simulink model "GDFLIB_FilterIIR2_BAM_FLT"  (Simulink 8.3)
settings: Solver=ode45  StartTime=0.0  StopTime=10.0  RelTol=1e-3
undefined symbols (not defined in the file): fltA1, fltA2, fltB0, fltB1, fltB2
settings Model: Creator=B17364  LastModifiedBy=B17364
settings OptimizationCC: ExpressionDepthLimit=2147483647
settings DebuggingCC: FcnCallInpInsideContextMsg=UseLocalSettings  StrictBusMsg=Warning

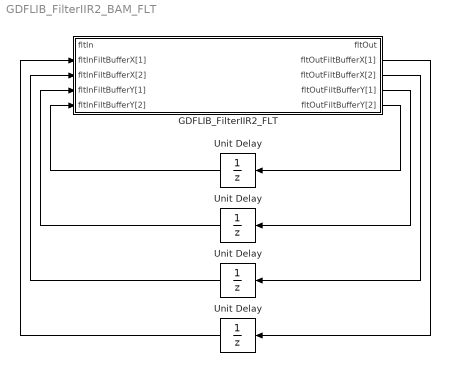
== system GDFLIB_FilterIIR2_BAM_FLT ==
  " Unit Delay" : UnitDelay  SampleTime=-1
  " Unit Delay " : UnitDelay  SampleTime=-1
  GDFLIB_FilterIIR2_FLT : Subsystem  mask(GDFLIB_FilterIIR2){fltB0=fltB0, fltB1=fltB1, fltB2=fltB2, fltA1=fltA1, fltA2=fltA2}
      mask help: Bit accurate model of direct form I second order IIR filter. All parameters as well as input and output are in single precision floating data format.
      mask init:
      | pos = get_param(gcb, 'Position');width = pos(3) - pos(1); height = pos(4) - pos(2);tX=width/2;tY=height*0.9;
      mask Display: color('black');port_label('input',1,'fltIn');port_label('input',2,'fltInFiltBufferX[1]');port_label('input',3,'fltInFiltBufferX[2]');port_label('input',4,'fltInFiltBufferY[1]');port_label('input',5,'fltInFiltBufferY[2]');port_label('output',1,'fltOut');port_label('output',2,'fltOutFiltBufferX[1]');port_label('output',3,'fltOutFiltBufferX[2]');port_label('output',4,'fltOutFiltBufferY[1]');port_label('output',5,'fltOutFiltBufferY[2]');color('black');disp('GDFLIB_FilterIIR2_FLT');color('blue');text(tX,tY, 'BAM', 'horizontalAlignment', 'center');
  Unit Delay : UnitDelay  SampleTime=-1
  "Unit Delay " : UnitDelay  SampleTime=-1
  wires:
  GDFLIB_FilterIIR2_FLT/5(fltOutFiltBufferY[2]) -> Unit Delay/1
  Unit Delay/1 -> GDFLIB_FilterIIR2_FLT/5(fltInFiltBufferY[2])
  GDFLIB_FilterIIR2_FLT/4(fltOutFiltBufferY[1]) -> "Unit Delay "/1
  "Unit Delay "/1 -> GDFLIB_FilterIIR2_FLT/4(fltInFiltBufferY[1])
  GDFLIB_FilterIIR2_FLT/3(fltOutFiltBufferX[2]) -> " Unit Delay"/1
  " Unit Delay"/1 -> GDFLIB_FilterIIR2_FLT/3(fltInFiltBufferX[2])
  GDFLIB_FilterIIR2_FLT/2(fltOutFiltBufferX[1]) -> " Unit Delay "/1
  " Unit Delay "/1 -> GDFLIB_FilterIIR2_FLT/2(fltInFiltBufferX[1])

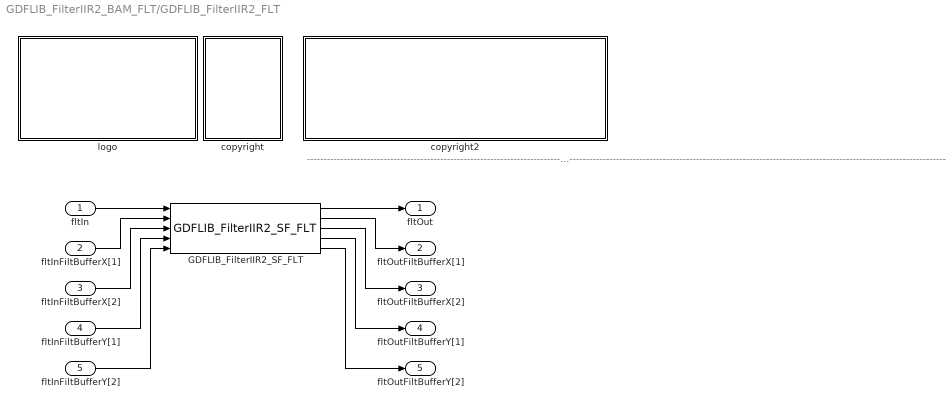
== system GDFLIB_FilterIIR2_BAM_FLT/GDFLIB_FilterIIR2_FLT ==
  note: ---------------------------------------------------------------------------------------------------------------------------------------------------------------------------------------------------
  fltIn : Inport
  fltInFiltBufferX[1] : Inport  Port=2
  fltInFiltBufferX[2] : Inport  Port=3
  fltInFiltBufferY[1] : Inport  Port=4
  fltInFiltBufferY[2] : Inport  Port=5
  GDFLIB_FilterIIR2_SF_FLT : S-Function  FunctionName=GDFLIB_FilterIIR2_SF_FLT  Parameters=fltB0,fltB1,fltB2,fltA1,fltA2  EnableBusSupport=off
  copyright : Subsystem
      mask Display:
      | text(10,90,'FILE:');text(10,75,'DESRIPTION:')
      | text(10,60,'COPYRIGHT:')
      | text(10,45,'VERSION:')
      | text(10,30,'DATE:')
      | text(10,15,'AUTHOR:')
  copyright2 : Subsystem
      mask Display:
      | text(10,90,'GDFLIB_FilterIIR2_BAM_FLT.mdl');text(10,75,'Direct form I second order IIR filter.');text(10,60,'Freescale')
      | text(10,45,'0.1');text(10,30,'08-Apr-2014');text(10,15,'');
  logo : Subsystem
      mask Display: image(imread('logo.jpg'))
  fltOut : Outport
  fltOutFiltBufferX[1] : Outport  Port=2
  fltOutFiltBufferX[2] : Outport  Port=3
  fltOutFiltBufferY[1] : Outport  Port=4
  fltOutFiltBufferY[2] : Outport  Port=5
  wires:
  fltIn/1 -> GDFLIB_FilterIIR2_SF_FLT/1
  GDFLIB_FilterIIR2_SF_FLT/1 -> fltOut/1
  fltInFiltBufferX[1]/1 -> GDFLIB_FilterIIR2_SF_FLT/2
  fltInFiltBufferX[2]/1 -> GDFLIB_FilterIIR2_SF_FLT/3
  fltInFiltBufferY[1]/1 -> GDFLIB_FilterIIR2_SF_FLT/4
  fltInFiltBufferY[2]/1 -> GDFLIB_FilterIIR2_SF_FLT/5
  GDFLIB_FilterIIR2_SF_FLT/2 -> fltOutFiltBufferX[1]/1
  GDFLIB_FilterIIR2_SF_FLT/3 -> fltOutFiltBufferX[2]/1
  GDFLIB_FilterIIR2_SF_FLT/4 -> fltOutFiltBufferY[1]/1
  GDFLIB_FilterIIR2_SF_FLT/5 -> fltOutFiltBufferY[2]/1

== system GDFLIB_FilterIIR2_BAM_FLT/GDFLIB_FilterIIR2_FLT/copyright ==

== system GDFLIB_FilterIIR2_BAM_FLT/GDFLIB_FilterIIR2_FLT/copyright2 ==

== system GDFLIB_FilterIIR2_BAM_FLT/GDFLIB_FilterIIR2_FLT/logo ==
